simulink model "HANcoder_E407_Local_Time_Ticks"  (R2018b)
settings: Solver=FixedStepDiscrete  StartTime=0.0  StopTime=1  FixedStep=0.01  RelTol=1e-3
PreLoadFcn:
  | librarySetup
  | eval([bdroot,'_startup']) %Calling [modelName]_startup.m
values from neighbouring files (symbols this model uses):
  HANtuneOverride = Simulink.Parameter    [HANcoder_E407_Local_Time_Ticks_startup.m]
libraries: HANcoder_STM32_Target x14, simulink x2, simulink_extras x1
CloseFcn:
  | rtwprivate ssgencode ModelCloseRequest mytest
settings Model: Creator=Jason van Kolfschoten  LastModifiedBy=Diego
settings SolverCC: PositivePriorityOrder=on
settings DataIOCC: LimitDataPoints=on  SaveFormat=Array  SignalLoggingSaveFormat=ModelDataLogs  SaveOutput=off  SaveTime=off
settings OptimizationCC: BlockReduction=off  DefaultParameterBehavior=Inlined  InlineInvariantSignals=on  ExpressionDepthLimit=2147483647  StateBitsets=on  DataBitsets=on  ZeroExternalMemoryAtStartup=off  ZeroInternalMemoryAtStartup=off  InitFltsAndDblsToZero=on  NoFixptDivByZeroProtection=on  EfficientFloat2IntCast=on  LifeSpan=inf
settings DebuggingCC: SaveWithDisabledLinksMsg=none  SaveWithParameterizedLinksMsg=none  CheckSSInitialOutputMsg=off  UnderspecifiedInitializationDetection=Classic  MergeDetectMultiDrivingBlocksExec=none  SignalResolutionControl=TryResolveAll  SolverPrmCheckMsg=warning  InheritedTsInSrcMsg=none  MultiTaskDSMMsg=warning  MultiTaskCondExecSysMsg=none  ParameterPrecisionLossMsg=none  FcnCallInpInsideContextMsg=warning  StateNameClashWarn=warning  SFUnexpectedBacktrackingDiag=warning  SFNoUnconditionalDefaultTransitionDiag=warning  SFExecutionAtInitializationDiag=none
settings HardwareCC: ProdBitPerPointer=32  ProdBitPerSizeT=32  ProdBitPerPtrDiffT=32  ProdLargestAtomicFloat=None  ProdIntDivRoundTo=Undefined  ProdWordSize=32  ProdHWDeviceType=Generic->32-bit Embedded Processor  TargetEndianess=LittleEndian  TargetHWDeviceType=Infineon->TriCore
settings ModelReferenceCC: PropagateSignalLabelsOutOfModel=off
settings SFSimCC: SimUseLocalCustomCode=off  MATLABDynamicMemAlloc=off
settings RTWCC: SystemTargetFile=ert.tlc  MakeCommand=make_rtw SHELL= HANcoder_PORTABLE=1 HANcoder_BOOTLOADER=1  TemplateMakefile=STM32_E407_gcc.tmf  Description=Real-Time Workshop Embedded Coder (no auto configuration)  RTWUseLocalCustomCode=off
settings CodeAppCC: ForceParamTrailComments=on  IgnoreCustomStorageClasses=off  SimulinkDataObjDesc=on  CustomSymbolStrGlobalVar=rt$N$M  CustomSymbolStrType=$N$M  CustomSymbolStrFcn=$N$M$F  CustomSymbolStrMacro=$N$M  InsertBlockDesc=on  StateflowObjectComments=on  InternalIdentifier=Classic
settings ERTTargetCC: TargetFcnLib=ansi_tfl_tmw.mat  MultiwordLength=2048  IncludeMdlTerminateFcn=off  SuppressErrorStatus=on  SupportNonFinite=off  GenerateASAP2=on  InlinedParameterPlacement=NonHierarchical  ERTCustomFileTemplate=example_file_process.tlc  ConvertIfToSwitch=off  SuppressUnreachableDefaultCases=off
settings ConfigComp: CovMetricSettings=dw  CovHtmlReporting=on  CovSaveCumulativeToWorkspaceVar=on  CovSaveSingleToWorkspaceVar=on  CovExternalEMLEnable=off  DVMaxProcessTime=600  DVDisplayUnsatisfiableObjectives=on  DVAutomaticStubbing=off  DVModelCoverageObjectives=MCDC  DVMaxTestCaseSteps=500  DVTestSuiteOptimization=CombinedObjectives  DVDetectActiveLogic=on  DVSaveHarnessModel=on

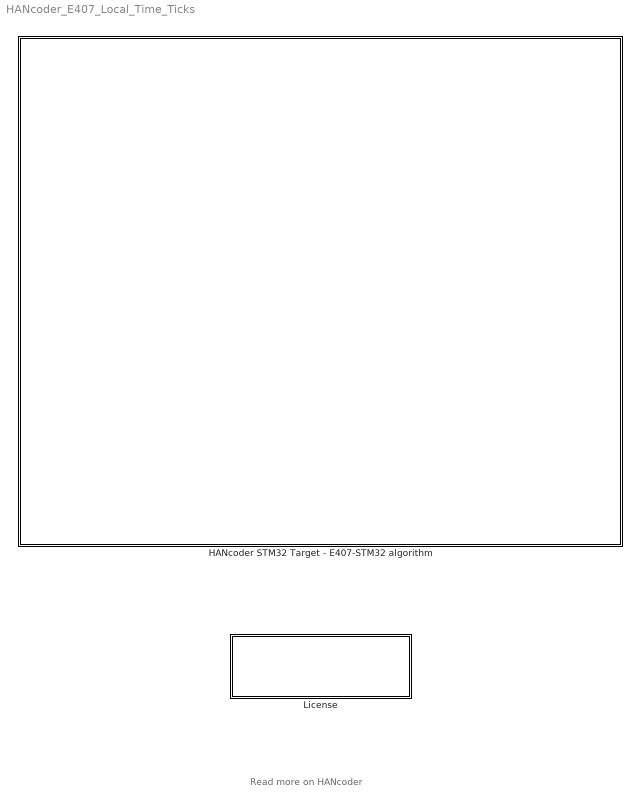
== system HANcoder_E407_Local_Time_Ticks ==
  note: Read more on HANcoder
  HANcoder STM32 Target - E407-STM32 algorithm : Subsystem  mask(TopLevelSubsystem){}
      settings: CopyFcn=HANcoderChecks('Copy');  NameChangeFcn=HANcoderChecks('NameChangeE407');  MoveFcn=HANcoderChecks('MoveE407');
      mask Display: image(imread('STM32_E407_HAN.jpg'))
  License : Subsystem  mask(License){}
      settings: NameChangeFcn=HANcoderChecks('NameChangeLicenseBlock');  OpenFcn=winopen('License.pdf')  MoveFcn=HANcoderChecks('MoveLicenseBlock');
      mask Display: disp(['End-User License Agreement\n','please read before use']);

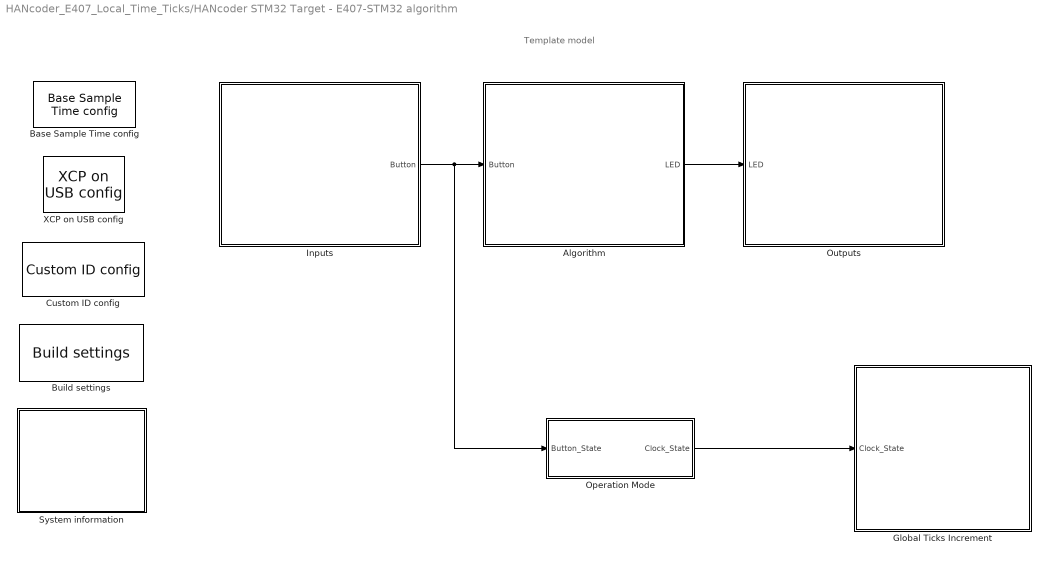
== system HANcoder_E407_Local_Time_Ticks/HANcoder STM32 Target - E407-STM32 algorithm ==
  note: Template model
  Algorithm : Subsystem
  Base Sample Time config : HANcoder_STM32_Target/STM32-E407/System Config/Base Sample Time config  Tag=HANcoder_TARGET_STM32_E407  Description=HANcoder Target STM32-E407 blockset version 0.5  baseSampleTime=10  extraStack=0
      settings: SourceProductName=HANcoder STM32 Target
  Build settings : HANcoder_STM32_Target/STM32-E407/System Config/Build settings  Tag=HANcoder_TARGET_STM32_E407  AutoASAP2add=on  AutoFlash=USB
      settings: SourceProductName=HANcoder STM32 Target
  Custom ID config : HANcoder_STM32_Target/STM32-E407/System Config/Custom ID config  Tag=HANcoder_TARGET_STM32_E407  softID=softwareID  softNUM=1
      settings: SourceProductName=HANcoder STM32 Target
  Global Ticks Increment : Subsystem
  Inputs : Subsystem
  Operation Mode : Subsystem
  Outputs : Subsystem
  System information : Subsystem
  XCP on USB config : HANcoder_STM32_Target/STM32-E407/System Config/XCP on USB config  Tag=HANcoder_TARGET_STM32_E407
      settings: SourceProductName=HANcoder STM32 Target
  wires:
  Algorithm/1(LED) -> Outputs/1(LED)
  Operation Mode/1(Clock_State) -> Global Ticks Increment/1(Clock_State)
  Inputs/1(Button) -> Operation Mode/1(Button_State), Algorithm/1(Button)

== system HANcoder_E407_Local_Time_Ticks/License ==

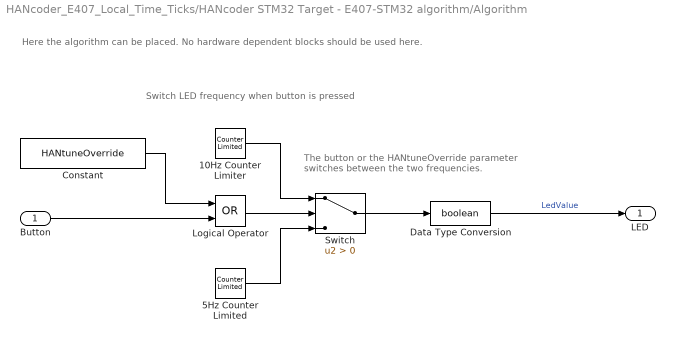
== system HANcoder_E407_Local_Time_Ticks/HANcoder STM32 Target - E407-STM32 algorithm/Algorithm ==
  note: The button or the HANtuneOverride parameter
      | switches between the two frequencies.
  note: Here the algorithm can be placed. No hardware dependent blocks should be used here.
  note: Switch LED frequency when button is pressed
  Button : Inport
  10Hz Counter Limiter : simulink/Sources/Counter Limited  uplimit=1  tsamp=0.1
  5Hz Counter Limited : simulink/Sources/Counter Limited  uplimit=1  tsamp=0.2
  Constant : Constant  Value=HANtuneOverride  OutDataTypeStr=boolean
  Data Type Conversion : DataTypeConversion  OutDataTypeStr=boolean
  Logical Operator : Logic  Operator=OR  AllPortsSameDT=off  OutDataTypeStr=boolean
  Switch : Switch  Criteria=u2 > Threshold
  LED : Outport
  wires:
  Data Type Conversion/1 -> LED/1  "LedValue"
  5Hz Counter Limited/1 -> Switch/3
  Switch/1 -> Data Type Conversion/1
  Button/1 -> Logical Operator/2
  Logical Operator/1 -> Switch/2
  Constant/1 -> Logical Operator/1
  10Hz Counter Limiter/1 -> Switch/1

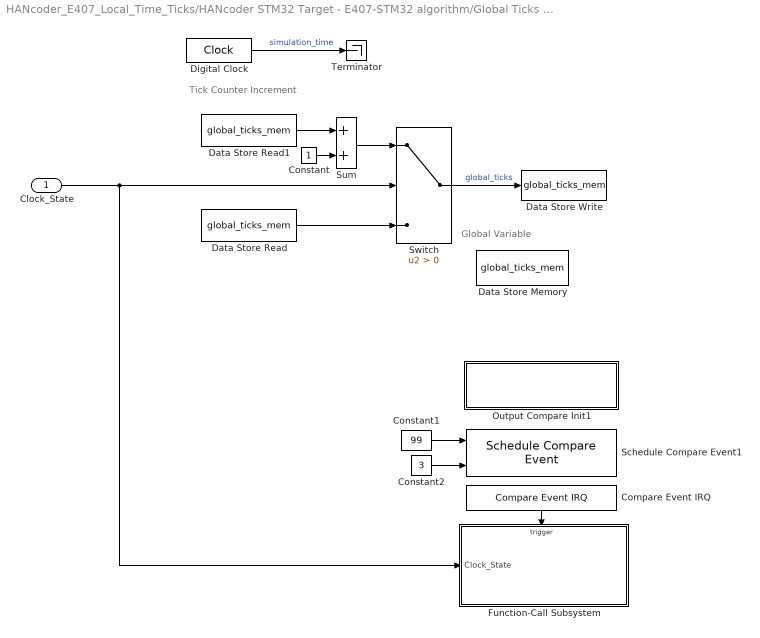
== system HANcoder_E407_Local_Time_Ticks/HANcoder STM32 Target - E407-STM32 algorithm/Global Ticks Increment ==
  note: Tick Counter Increment
  note: Global Variable
  Clock_State : Inport
  Compare Event IRQ : HANcoder_STM32_Target/STM32-E407/Timer Outputs/Compare Event IRQ  Tag=HANcoder_TARGET_STM32_E407  pin=TIM4 - CON PD - 15 - 5V Tolerant
      settings: SourceProductName=HANcoder STM32 Target
  Constant : Constant
  Constant1 : Constant  Value=99  OutDataTypeStr=uint16
  Constant2 : Constant  Value=3  OutDataTypeStr=uint8
  Data Store Memory : DataStoreMemory  DataStoreName=global_ticks_mem  ReadBeforeWriteMsg=warning  WriteAfterWriteMsg=warning  WriteAfterReadMsg=warning  ShowAdditionalParam=off
  Data Store Read : DataStoreRead  DataStoreName=global_ticks_mem
  Data Store Read1 : DataStoreRead  DataStoreName=global_ticks_mem
  Data Store Write : DataStoreWrite  DataStoreName=global_ticks_mem
  Digital Clock : DigitalClock  SampleTime=0.01
  Function-Call Subsystem : Subsystem  TreatAsAtomicUnit=on
  Output Compare Init1 : Subsystem  Tag=HANcoder_TARGET_STM32_E407  AncestorBlock=HANcoder_STM32_Target/STM32-E407/Timer Outputs/Output Compare Init  mask(Output Compare Init){moduleID=TIM4 - CON PD - 15 & 16 &n/a & n/a, frequency=1000000, enableIRQoutput=off}
      mask prompts: moduleID "Timer module"; frequency "Frequency (free running counter) [Hz]"; enableIRQoutput "Enable IRQ output"
      mask help:
      | Function
      | ========
      | Initializes the timer module to allow output compare functionality on the
      | module's channels.
      |
      | Parameters
      | ==========
      | Timer Module:
      |   Selects the timer module.
      |
      | Frequency:
      |   Frequency at which the 16-bit free running counter counts.
      |
      | Enable IRQ output
      |   Controls whether or not the IRQ output is available.
      |
      | Outport
      | =======
      | IRQ
      |   Allows connection of a function call subsystem for the free running
      |   counter overflow event.
      mask init:
      | moduleIDInfoStr = sfcn_timeout_init_mcb(2, moduleID, frequency, enableIRQoutput);
      settings: CopyFcn=sfcn_timeout_init_chk();  MoveFcn=drawLogos
      mask Help: web('sfcn_timeout_init.html');
      mask TypeOptions moduleID: TIM1 - CON PE - 12 & 14 & 16 & 17 | TIM2 - CON4 - D13 & n/a & n/a & n/a | TIM3 - CON4 - D12 & D11 & n/a & n/a | TIM4 - CON PD - 15 & 16 &n/a & n/a | TIM8 - UEXT - 3 & 4 & n/a & n/a | TIM9 - CON3 - D4 & D5 or PE - 8 & 9 | TIM10 - CON2 - A1 or CON PF - 9 | TIM11 - CON2 - A2 or CON PF - 10 | TIM13 - CON2 - A3 or CON PF - 11 | TIM14 - CON2 - A4 or CON PF - 12
      mask Callback moduleID: sfcn_timeout_init_chk();
      mask Display: fprintf('Output Compare Init\n%s', moduleIDInfoStr);patch([135 141 141],[8 14 2],[1 0 0]);patch([143 143 149],[14 2 8],[0 0 0.35]);
  Schedule Compare Event1 : HANcoder_STM32_Target/STM32-E407/Timer Outputs/Schedule Compare Event  Tag=HANcoder_TARGET_STM32_E407  pin=TIM4 - CON PD - 15 - 5V Tolerant  tsamp=-1
      settings: SourceProductName=HANcoder STM32 Target
  Sum : Sum
  Switch : Switch  Criteria=u2 > Threshold
  Terminator : Terminator
  wires:
  Clock_State/1 -> Function-Call Subsystem/1(Clock_State), Switch/2
  Digital Clock/1 -> Terminator/1  "simulation_time"
  Switch/1 -> Data Store Write/1  "global_ticks"
  Data Store Read/1 -> Switch/3
  Sum/1 -> Switch/1
  Data Store Read1/1 -> Sum/1
  Constant/1 -> Sum/2
  Constant2/1 -> Schedule Compare Event1/2
  Constant1/1 -> Schedule Compare Event1/1
  Compare Event IRQ/1 -> Function-Call Subsystem/Trigger

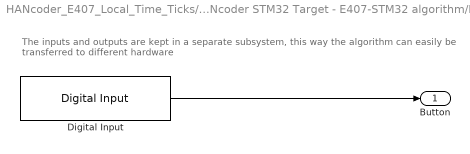
== system HANcoder_E407_Local_Time_Ticks/HANcoder STM32 Target - E407-STM32 algorithm/Inputs ==
  note: The inputs and outputs are kept in a separate subsystem, this way the algorithm can easily be transferred to different hardware
  Digital Input : HANcoder_STM32_Target/STM32-E407/Digital Inputs/Digital Input  Tag=HANcoder_TARGET_STM32_E407  pinID=WKUP button  config=Pulldown  tsamp=-1
      settings: SourceProductName=HANcoder STM32 Target
  Button : Outport
  wires:
  Digital Input/1 -> Button/1

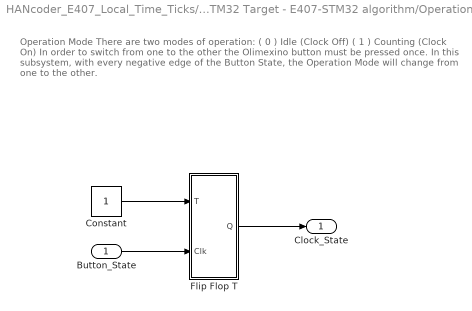
== system HANcoder_E407_Local_Time_Ticks/HANcoder STM32 Target - E407-STM32 algorithm/Operation Mode ==
  note: Operation Mode
      | There are two modes of operation:
      | ( 0 ) Idle (Clock Off)
      | ( 1 ) Counting (Clock On)
      | In order to switch from one to the other the Olimexino button
      | must be pressed once. In this subsystem, with every negative
      | edge of the Button State, the Operation Mode will change from
      | one to the other.
  Button_State : Inport
  Constant : Constant  OutDataTypeStr=boolean
  Flip Flop T : Subsystem
  Clock_State : Outport
  wires:
  Constant/1 -> Flip Flop T/1(T)
  Button_State/1 -> Flip Flop T/2(Clk)
  Flip Flop T/1(Q) -> Clock_State/1

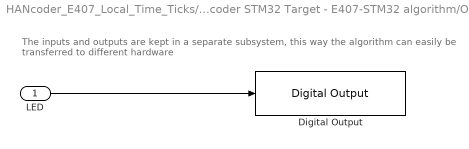
== system HANcoder_E407_Local_Time_Ticks/HANcoder STM32 Target - E407-STM32 algorithm/Outputs ==
  note: The inputs and outputs are kept in a separate subsystem, this way the algorithm can easily be transferred to different hardware
  LED : Inport
  Digital Output : HANcoder_STM32_Target/STM32-E407/Digital Outputs/Digital Output  Tag=HANcoder_TARGET_STM32_E407  pinID=LED  config=Push pull  tsamp=-1
      settings: SourceProductName=HANcoder STM32 Target
  wires:
  LED/1 -> Digital Output/1

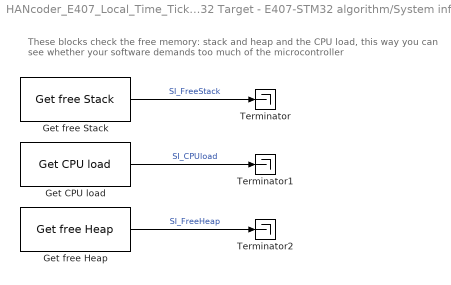
== system HANcoder_E407_Local_Time_Ticks/HANcoder STM32 Target - E407-STM32 algorithm/System information ==
  note: These blocks check the free memory: stack and heap and the CPU load,
      | this way you can see whether your software demands too much of the microcontroller
  Get CPU load : HANcoder_STM32_Target/STM32-E407/System Management/Get CPU load  Tag=HANcoder_TARGET_STM32_E407  mode=Current CPU load  tsamp=-1
      settings: SourceProductName=HANcoder STM32 Target
  Get free Heap : HANcoder_STM32_Target/STM32-E407/System Management/Get free Heap  Tag=HANcoder_TARGET_STM32_E407  tsamp=-1
      settings: SourceProductName=HANcoder STM32 Target
  Get free Stack : HANcoder_STM32_Target/STM32-E407/System Management/Get free Stack  Tag=HANcoder_TARGET_STM32_E407  taskIdx=Application Control Task  tsamp=-1
      settings: SourceProductName=HANcoder STM32 Target
  Terminator : Terminator
  Terminator1 : Terminator
  Terminator2 : Terminator
  wires:
  Get CPU load/1 -> Terminator1/1  "SI_CPUload"
  Get free Stack/1 -> Terminator/1  "SI_FreeStack"
  Get free Heap/1 -> Terminator2/1  "SI_FreeHeap"

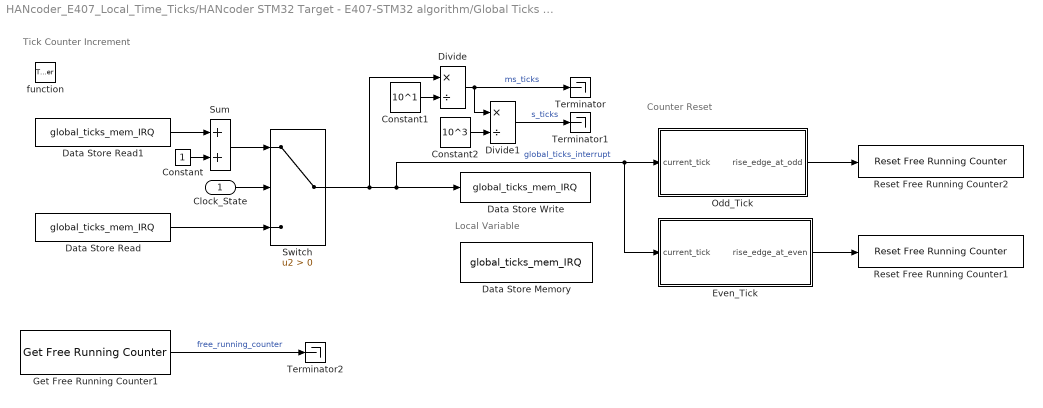
== system HANcoder_E407_Local_Time_Ticks/HANcoder STM32 Target - E407-STM32 algorithm/Global Ticks Increment/Function-Call Subsystem ==
  note: Counter Reset
  note: Tick Counter Increment
  note: Local Variable
  Clock_State : Inport
  function : TriggerPort  TriggerType=function-call  VariantControl=Variant
  Constant : Constant
  Constant1 : Constant  Value=10^1
  Constant2 : Constant  Value=10^3
  Data Store Memory : DataStoreMemory  DataStoreName=global_ticks_mem_IRQ  ReadBeforeWriteMsg=warning  WriteAfterWriteMsg=warning  WriteAfterReadMsg=warning  ShowAdditionalParam=off
  Data Store Read : DataStoreRead  DataStoreName=global_ticks_mem_IRQ
  Data Store Read1 : DataStoreRead  DataStoreName=global_ticks_mem_IRQ
  Data Store Write : DataStoreWrite  DataStoreName=global_ticks_mem_IRQ
  Divide : Product  Inputs=*/
  Divide1 : Product  Inputs=*/
  Even_Tick : Stateflow chart  TreatAsAtomicUnit=on
  Get Free Running Counter1 : HANcoder_STM32_Target/STM32-E407/Timer Outputs/Get Free Running Counter  Tag=HANcoder_TARGET_STM32_E407  moduleID=TIM4 - CON PD - 15 & 16 &n/a & n/a  tsamp=-1
      settings: SourceProductName=HANcoder STM32 Target
  Odd_Tick : Stateflow chart  TreatAsAtomicUnit=on
  Reset Free Running Counter1 : HANcoder_STM32_Target/STM32-E407/Timer Outputs/Reset Free Running Counter  Tag=HANcoder_TARGET_STM32_E407  moduleID=TIM4 - CON PD - 15 & 16 &n/a & n/a
      settings: SourceProductName=HANcoder STM32 Target
  Reset Free Running Counter2 : HANcoder_STM32_Target/STM32-E407/Timer Outputs/Reset Free Running Counter  Tag=HANcoder_TARGET_STM32_E407  moduleID=TIM4 - CON PD - 15 & 16 &n/a & n/a
      settings: SourceProductName=HANcoder STM32 Target
  Sum : Sum
  Switch : Switch  Criteria=u2 > Threshold
  Terminator : Terminator
  Terminator1 : Terminator
  Terminator2 : Terminator
  wires:
  Constant/1 -> Sum/2
  Switch/1 -> Data Store Write/1, Even_Tick/1(current_tick), Odd_Tick/1(current_tick), Divide/1  "global_ticks_interrupt"
  Clock_State/1 -> Switch/2
  Data Store Read1/1 -> Sum/1
  Sum/1 -> Switch/1
  Data Store Read/1 -> Switch/3
  Constant1/1 -> Divide/2
  Divide/1 -> Divide1/1, Terminator/1  "ms_ticks"
  Divide1/1 -> Terminator1/1  "s_ticks"
  Constant2/1 -> Divide1/2
  Get Free Running Counter1/1 -> Terminator2/1  "free_running_counter"
  Even_Tick/1(rise_edge_at_even) -> Reset Free Running Counter1/Trigger
  Odd_Tick/1(rise_edge_at_odd) -> Reset Free Running Counter2/Trigger

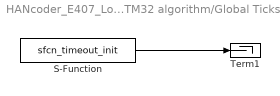
== system HANcoder_E407_Local_Time_Ticks/HANcoder STM32 Target - E407-STM32 algorithm/Global Ticks Increment/Output Compare Init1 ==
  S-Function : S-Function  FunctionName=sfcn_timeout_init  SFunctionDeploymentMode=off  EnableBusSupport=off
  Term1 : Terminator
  wires:
  S-Function/1 -> Term1/1

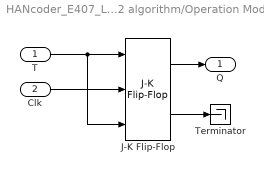
== system HANcoder_E407_Local_Time_Ticks/HANcoder STM32 Target - E407-STM32 algorithm/Operation Mode/Flip Flop T ==
  T : Inport
  Clk : Inport  Port=2
  J-K Flip-Flop : simulink_extras/Flip Flops/J-K Flip-Flop  initial_condition=0
      settings: SourceProductName=Simulink
  Terminator : Terminator
  Q : Outport
  wires:
  J-K Flip-Flop/2 -> Terminator/1
  T/1 -> J-K Flip-Flop/3, J-K Flip-Flop/1
  J-K Flip-Flop/1 -> Q/1
  Clk/1 -> J-K Flip-Flop/2

== stateflow chart HANcoder_E407_Local_Time_Ticks/HANcoder STM32 Target - E407-STM32 algorithm/Global Ticks Increment/Function-Call Subsystem/Even_Tick ==
  settings: initializeOutput=1
  state Even_tick
    if (mod(current_tick,2)==0)
    active_flag = 1;
    end
  state Rise_edge
    send(rise_edge_at_even)
  (default) -> Even_tick
  Even_tick -> Rise_edge : [active_flag == 1]
  data: current_tick input; active_flag local =0
  events: rise_edge_at_even output EITHER_EDGE_EVENT

== stateflow chart HANcoder_E407_Local_Time_Ticks/HANcoder STM32 Target - E407-STM32 algorithm/Global Ticks Increment/Function-Call Subsystem/Odd_Tick ==
  settings: initializeOutput=1
  state Odd_tick
    if (mod(current_tick,2)==1)
    active_flag = 1;
    end
  state Rise_edge
    send(rise_edge_at_odd)
  (default) -> Odd_tick
  Odd_tick -> Rise_edge : [active_flag == 1]
  data: current_tick input; active_flag local =0
  events: rise_edge_at_odd output EITHER_EDGE_EVENT
